simulink model "CubeX"  (R2016b)
settings: Solver=FixedStepAuto  StartTime=0.0  StopTime=10.0  RelTol=1e-3
values from neighbouring files (symbols this model uses):
  A = [0 0 0 0 0 0 0 0 0 0 283.190307038 0 ... (36 elements, 6x6)]    [K_lqr_3D.mat]
  C = [1 0 0 0 0 0 0 1 0 0 0 0 ... (36 elements, 6x6)]    [K_lqr_3D.mat]
  controller =     [K_lqr_3D.mat]
  deg_ = 0.0174532925199    [K_lqr_3D.mat]
  g = 9.81    [K_lqr_3D.mat]
  imu =     [K_lqr_3D.mat]
  K_lqr = [204.402503892 25.7626324054]    [K_lqr_3D.mat]
undefined symbols (not defined in the file or in its folder): CPHA_1Edge, CPOL_Low, Duplex, FirstBit_MSB, Full, Link, LQFP100, ST, STM32F407VG, STM32F4DISCOVERY
libraries: simulink x22, stm32f4_spi_lib x4, stm32f4_io_lib x2, stm32f4_adc_lib x1, cube_lib x1, stm32f4_device_config_lib x1, BC_USB x1
(part 3 of 3)

== matlab function CubeX/SPI3 get Data4/Take away Sensor fail reading if two bad in raw2 ==
  data: y output; new input; old input
function y = fcn(new, old)
%#codegen
if(new > -257 && new < -200)
   y = old;
else
    y = new;
end

== matlab function CubeX/SPI3 get Data4/Take away Sensor fail reading2 ==
  data: y output; new input; old input
function y = fcn(new, old)
%#codegen
if(new > -257 && new < -200)
   y = old;
else
    y = new;
end
